simulink library "sm_motor_grader_lib"  (R2026a)
settings: Solver=VariableStepAuto
undefined symbols (not defined in the file): activeTestCmds, Art, Center, Circle, Driver, HMPST, LiftL, LiftR, LnL, LnR, Loads, Maneuver, motGradParams, Pin, RFL, RFR, RRL, RRR, SceneData, Side, Sphere, StrL, StrR, Tilt, X, Y, Z
libraries: sm_lib x219, nesl_utility x134, fl_lib x53, $bdroot x24, cvt_powertrain_lib x6, simulink_extras x5, grid_element x4, simulink x3, cvt_powertrain_lib_vnts x3, Driver_Long_Lat_Stanley x1, Maneuver_Get_Pose x1, SignalEditorBlockLib x1
(part 1 of 13)
Description:
  | Copyright 2025-2026 The MathWorks, Inc.
settings Model: Creator=smiller  LastModifiedBy=smiller

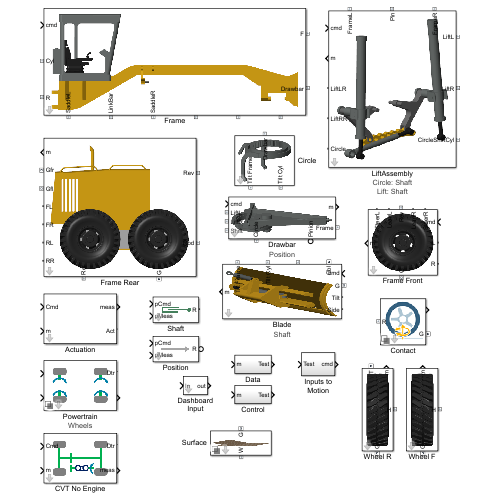
[thumbnail: Simulink's stored preview of the top-level diagram]
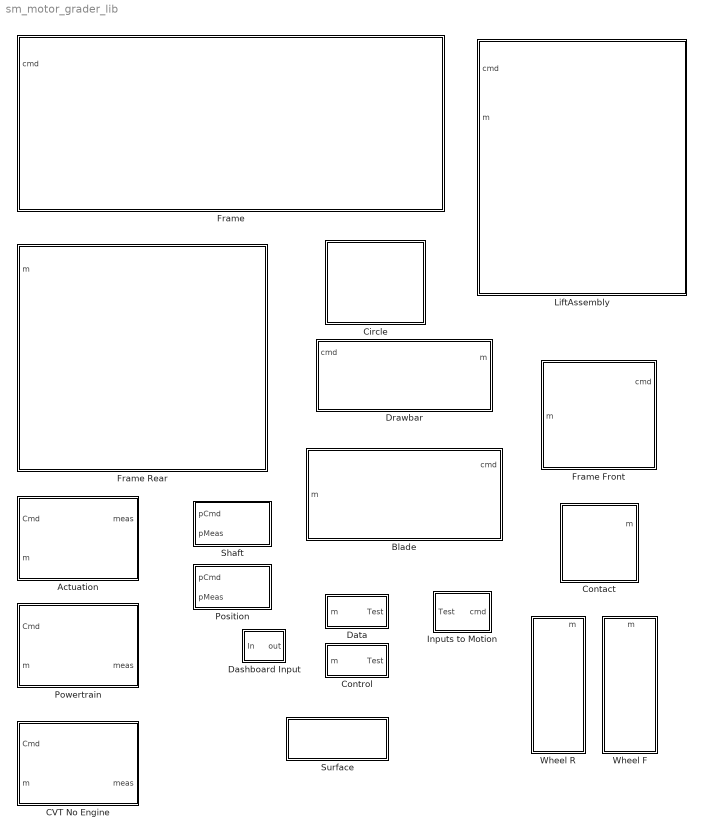
== system sm_motor_grader_lib ==
  Actuation : Subsystem  VariantControl=Actuation  mask{popup_actuator_model=Position, popup_actuator_model_lift=Shaft}
      mask prompts: popup_actuator_model "Actuation Mode"; popup_actuator_model_lift "Actuation Mode Lift"
      mask init:
      | bh = gcb;
      | modestr = get_param(bh,'popup_actuator_model');
      | set_param([bh '/Actuator Tilt'],'LabelModeActiveChoice',modestr)
      | set_param([bh '/Actuator Shift'],'LabelModeActiveChoice',modestr)
      | set_param([bh '/Actuator Articulation'],'LabelModeActiveChoice',modestr)
      | set_param([bh '/Actuator Circle'],'LabelModeActiveChoice',modestr)
      | set_param([bh '/Actuator SteerL'],'LabelModeActiveChoice',modestr)
      | set_param([bh '/Actuator SteerR'],'LabelModeActiveChoice',modestr)
      | set_param([bh '/Actuator LeanL'],'LabelModeActiveChoice',modestr)
      | set_param([bh '/Actuator LeanR'],'LabelModeActiveChoice',modestr)
      | set_param([bh '/Actuator Pinion'],'LabelModeActiveChoice',modestr)
      | 
      | liftmodestr = get_param(bh,'popup_actuator_model_lift');
      | set_param([bh '/Actuator LiftL'],'LabelModeActiveChoice',liftmodestr)
      | set_param([bh '/Actuator LiftR'],'LabelModeActiveChoice',liftmodestr)
      mask TypeOptions popup_actuator_model: Position | Shaft
      mask TypeOptions popup_actuator_model_lift: Position | Shaft
  Blade : Subsystem  mask{popup_actuator_model=Shaft, popup_blade_ground_contact=Loads}
      mask prompts: popup_actuator_model "Actuation Mode"; popup_blade_ground_contact "Blade Ground Contact"
      mask init:
      | bh = gcb;
      | if(strcmp(get_param(bh,'popup_actuator_model'),'Shaft'))
      |     set_param([bh '/Tilt Actuator'],'popup_actuator_model','Shaft')
      |     set_param([bh '/Shift Actuator'],'popup_actuator_model','Shaft')
      | else
      |     set_param([bh '/Tilt Actuator'],'popup_actuator_model','Position')
      |     set_param([bh '/Shift Actuator'],'popup_actuator_model','Position')
      | end
      settings: AttributesFormatString=%<popup_actuator_model>  PortSchema="{\"entries\":[{\"content\":{\"sides\":[{\"content\":{\"connectorIds\":[\"In1\",\"LConn1\",\"LConn2\",\"LConn3\"]},\"type\":\"ConnectorPlacement.EquallySpacedRectSide\",\"uuid\":\"64dbd0ba-121a-468c-87f8-2fede28d7949\"},{\"content\":{\"connectorIds\":[\"Out1\"],\"side\":\"RIGHT\"},\"type\":\"ConnectorPlacement.EquallySpacedRectSide\",\"uuid\":\"d521fda1-87cd-4ba3-938c-38986a441e94\"},{\"content\":{\"connectorIds\":[\"LConn4\",\"LConn5\",\"LConn6\",\"LConn7\"],\"side\":\"TOP\"},\"type\":\"ConnectorPlacement.EquallySpacedRectSide\",\"uuid\":\"c03a1403-e105-4f6f-8c6b-d646839b846b\"}]},\"type\":\"ConnectorPlacement.EquallySpacedConnector\",\"uuid\":\"70598b05-b8b5-4d67-bbf4-55a5797dbb69\"}],\"packageUris\":[\"http://schema.mathworks.com/mf0/Connector/R2020b\"],\"version\":\"1.0\"}"
      mask TypeOptions popup_actuator_model: Position | Shaft
      mask TypeOptions popup_blade_ground_contact: Blade/popup_blade_ground_contact
      mask Display: image('sm_motor_grader_moldboard_IMAGE.png')
  CVT No Engine : Subsystem  VariantControl=CVT
      settings: PortSchema="{\"entries\":[{\"content\":{\"sides\":[{\"content\":{\"connectorIds\":[\"In1\",\"In2\"]},\"type\":\"ConnectorPlacement.EquallySpacedRectSide\",\"uuid\":\"b0ddd375-51b8-44b6-b073-16b56860cf73\"},{\"content\":{\"connectorIds\":[\"RConn1\",\"Out1\"],\"side\":\"RIGHT\"},\"type\":\"ConnectorPlacement.EquallySpacedRectSide\",\"uuid\":\"f6b94886-5d75-4a34-bd54-ed8eca8a2f91\"},{\"content\":{\"side\":\"TOP\"},\"type\":\"ConnectorPlacement.EquallySpacedRectSide\",\"uuid\":\"a9bdb5f3-5bc9-4293-95f7-be33271ad817\"}]},\"type\":\"ConnectorPlacement.EquallySpacedConnector\",\"uuid\":\"99647ee7-7b0f-4a9d-8234-cdeac05b9707\"}],\"packageUris\":[\"http://schema.mathworks.com/mf0/Connector/R2020b\"],\"version\":\"1.0\"}"
      mask Display: image('ssc_4whl_powertrain_cvt.png')
  Circle : Subsystem
      settings: PortSchema="{\"entries\":[{\"content\":{\"sides\":[{\"content\":{},\"type\":\"ConnectorPlacement.EquallySpacedRectSide\",\"uuid\":\"63ab4a23-8b89-415d-877f-feb881a061f1\"},{\"content\":{\"side\":\"RIGHT\"},\"type\":\"ConnectorPlacement.EquallySpacedRectSide\",\"uuid\":\"0092ed81-5b75-47ad-b9e7-41c464aec9e6\"},{\"content\":{\"connectorIds\":[\"LConn1\"],\"side\":\"TOP\"},\"type\":\"ConnectorPlacement.EquallySpacedRectSide\",\"uuid\":\"752d188f-c013-4e13-8b29-1d347d2a3863\"},{\"content\":{\"connectorIds\":[\"RConn1\",\"RConn2\"],\"side\":\"BOTTOM\"},\"type\":\"ConnectorPlacement.EquallySpacedRectSide\",\"uuid\":\"b80fa618-c4c3-4c2f-8b58-79928366cbe4\"}]},\"type\":\"ConnectorPlacement.EquallySpacedConnector\",\"uuid\":\"1b957d24-5c42-454c-a11d-5e6b523a4d4e\"}],\"packageUris\":[\"http://schema.mathworks.com/mf0/Connector/R2020b\"],\"version\":\"1.0\"}"
      mask Display: image('sm_motor_grader_circle_IMAGE.png')
  Contact : Subsystem  Variant=on  VariantControlMode=label  VariantControl=Sphere  LabelModeActiveChoice=Magic Formula
  Control : Subsystem  VariantControl=Control
  Dashboard Input : Subsystem  mask{upper_bound=0, lower_bound=motGradParams.articulation.lowerBound, U0=motGradParams.articulation.initPos, tfilt=0.1}
      mask prompts: upper_bound "Upper Bound"; lower_bound "Lower Bound"; U0 "SimulinkBlocks:simulink_extras:InitialInput_MP"; tfilt "Filter Constant"
      mask TypeOptions U0:
      | Transfer Fcn
      | (with initial outputs)/U0 | Transfer Fcn
      | (with initial outputs)/Y0
      mask DialogControl U0 Prompt: Initial input:
  Data : Subsystem  VariantControl=Data
  Drawbar : Subsystem  mask{popup_actuator_model=Position}
      mask prompts: popup_actuator_model "Actuation Mode"
      mask init:
      | bh = gcb;
      | if(strcmp(get_param(bh,'popup_actuator_model'),'Shaft'))
      |     set_param([bh '/Actuator'],'LabelModeActiveChoice','Shaft')
      | else
      |     set_param([bh '/Actuator'],'LabelModeActiveChoice','Position')
      | end
      settings: AttributesFormatString=%<popup_actuator_model>  PortSchema="{\"entries\":[{\"content\":{\"sides\":[{\"content\":{\"connectorIds\":[\"In1\",\"LConn1\",\"LConn2\",\"LConn3\"]},\"type\":\"ConnectorPlacement.EquallySpacedRectSide\",\"uuid\":\"7234e91a-ed4b-4098-8d23-6b77775b5b7f\"},{\"content\":{\"connectorIds\":[\"Out1\",\"RConn1\"],\"side\":\"RIGHT\"},\"type\":\"ConnectorPlacement.EquallySpacedRectSide\",\"uuid\":\"48f806ee-3ea7-460b-b9fa-1f56f5dd994a\"},{\"content\":{\"side\":\"TOP\"},\"type\":\"ConnectorPlacement.EquallySpacedRectSide\",\"uuid\":\"5b9f253b-2dbf-4601-908f-7111d138ba6e\"},{\"content\":{\"connectorIds\":[\"RConn2\",\"RConn3\"],\"side\":\"BOTTOM\"},\"type\":\"ConnectorPlacement.EquallySpacedRectSide\",\"uuid\":\"9be04b94-2c6d-44c4-9c03-8c052620d49b\"}]},\"type\":\"ConnectorPlacement.EquallySpacedConnector\",\"uuid\":\"9d0450f6-732d-46a7-b755-37fed4fce1e3\"}],\"packageUris\":[\"http://schema.mathworks.com/mf0/Connector/R2020b\"],\"version\":\"1.0\"}"
      mask TypeOptions popup_actuator_model: Position | Shaft
      mask Display: image('sm_motor_grader_drawbar_IMAGE.png')
  Frame : Subsystem
      settings: PortSchema="{\"entries\":[{\"content\":{\"sides\":[{\"content\":{\"connectorIds\":[\"In1\",\"LConn1\",\"LConn2\"]},\"type\":\"ConnectorPlacement.EquallySpacedRectSide\",\"uuid\":\"b4e4171d-0284-478f-93eb-e40a965869bd\"},{\"content\":{\"connectorIds\":[\"RConn1\",\"RConn2\"],\"side\":\"RIGHT\"},\"type\":\"ConnectorPlacement.EquallySpacedRectSide\",\"uuid\":\"a326bb83-43f6-4b0d-ba21-f055f0976929\"},{\"content\":{\"side\":\"TOP\"},\"type\":\"ConnectorPlacement.EquallySpacedRectSide\",\"uuid\":\"b7d1be37-3d49-41f6-8566-6d4da5b1cd99\"},{\"content\":{\"connectorIds\":[\"RConn3\",\"RConn4\",\"RConn5\",\"RConn6\",\"RConn7\",\"RConn8\"],\"side\":\"BOTTOM\"},\"type\":\"ConnectorPlacement.EquallySpacedRectSide\",\"uuid\":\"50e3951f-3737-46e1-aff9-2ccd4ba65e65\"}]},\"type\":\"ConnectorPlacement.EquallySpacedConnector\",\"uuid\":\"94325d30-52dd-4a6f-8a1a-f56bc213c0cf\"}],\"packageUris\":[\"http://schema.mathworks.com/mf0/Connector/R2020b\"],\"version\":\"1.0\"}"
      mask Display: image('sm_motor_grader_frameCab_IMAGE.png')
  Frame Front : Subsystem  mask{popup_actuator_model=Shaft, popup_ground_contact=Sphere}
      mask prompts: popup_actuator_model "Actuation Mode"; popup_ground_contact "Ground Contact"
      mask init:
      | bh = gcb;
      | if(strcmp(get_param(bh,'popup_actuator_model'),'Shaft'))
      |     set_param([bh '/Lean Cylinder L'],'popup_actuator_model','Shaft')
      |     set_param([bh '/Lean Cylinder R'],'popup_actuator_model','Shaft')
      |     set_param([bh '/Steer Cylinder L'],'popup_actuator_model','Shaft')
      |     set_param([bh '/Steer Cylinder R'],'popup_actuator_model','Shaft')
      | else
      |     set_param([bh '/Lean Cylinder L'],'popup_actuator_model','Position')
      |     set_param([bh '/Lean Cylinder R'],'popup_actuator_model','Position')
      |     set_param([bh '/Steer Cylinder L'],'popup_actuator_model','Position')
      |     set_param([bh '/Steer Cylinder R'],'popup_actuator_model','Position')
      | end
      settings: PortSchema="{\"entries\":[{\"content\":{\"sides\":[{\"content\":{\"connectorIds\":[\"In1\",\"LConn1\",\"LConn2\"]},\"type\":\"ConnectorPlacement.EquallySpacedRectSide\",\"uuid\":\"d719529f-17dc-4c69-a89e-e71c8b487632\"},{\"content\":{\"connectorIds\":[\"Out1\"],\"side\":\"RIGHT\"},\"type\":\"ConnectorPlacement.EquallySpacedRectSide\",\"uuid\":\"e7fa06bf-1a63-484a-b998-aaa1bdc34664\"},{\"content\":{\"connectorIds\":[\"LConn3\",\"LConn4\",\"LConn5\",\"LConn6\",\"LConn7\"],\"side\":\"TOP\"},\"type\":\"ConnectorPlacement.EquallySpacedRectSide\",\"uuid\":\"3b968ecd-8edf-4595-9577-41521836e52d\"},{\"content\":{\"connectorIds\":[\"RConn1\"],\"side\":\"BOTTOM\"},\"type\":\"ConnectorPlacement.EquallySpacedRectSide\",\"uuid\":\"998a1490-38ee-4f90-9f0c-64c247eb2ef3\"}]},\"type\":\"ConnectorPlacement.EquallySpacedConnector\",\"uuid\":\"66e6443c-e818-4a0b-88cc-b534e33fe9c1\"}],\"packageUris\":[\"http://schema.mathworks.com/mf0/Connector/R2020b\"],\"version\":\"1.0\"}"
      mask TypeOptions popup_actuator_model: Position | Shaft
      mask TypeOptions popup_ground_contact: Wheel FL/popup_ground_contact | Wheel FR/popup_ground_contact
      mask Display: image('sm_motor_grader_frameFront_IMAGE.png')
  Frame Rear : Subsystem  mask{popup_ground_contact=Sphere}
      mask prompts: popup_ground_contact "Ground Contact"
      settings: PortSchema="{\"entries\":[{\"content\":{\"sides\":[{\"content\":{\"connectorIds\":[\"LConn1\",\"LConn2\"]},\"type\":\"ConnectorPlacement.EquallySpacedRectSide\",\"uuid\":\"e776eb69-fe07-42f6-973c-e6579d9bb0af\"},{\"content\":{\"connectorIds\":[\"Out1\",\"RConn1\",\"RConn2\",\"RConn3\",\"RConn4\",\"RConn5\",\"RConn6\"],\"side\":\"RIGHT\"},\"type\":\"ConnectorPlacement.EquallySpacedRectSide\",\"uuid\":\"308f9881-db51-4dcf-ba81-b3094ed7176e\"},{\"content\":{\"side\":\"TOP\"},\"type\":\"ConnectorPlacement.EquallySpacedRectSide\",\"uuid\":\"d5cd9905-25fb-439a-a908-e078aef10600\"},{\"content\":{\"connectorIds\":[\"RConn7\",\"RConn8\"],\"side\":\"BOTTOM\"},\"type\":\"ConnectorPlacement.EquallySpacedRectSide\",\"uuid\":\"fcfd5f0a-595a-4c14-8789-0bf7c20d2a5f\"}]},\"type\":\"ConnectorPlacement.EquallySpacedConnector\",\"uuid\":\"05355ae5-5c0f-4ba9-8d92-15da5bd4be6c\"}],\"packageUris\":[\"http://schema.mathworks.com/mf0/Connector/R2020b\"],\"version\":\"1.0\"}"
      mask TypeOptions popup_ground_contact: Wheel FL/popup_ground_contact | Wheel FR/popup_ground_contact | Wheel RL/popup_ground_contact | Wheel RR/popup_ground_contact
      mask Display: image('sm_motor_grader_frameRear_IMAGE.png')
  Inputs to Motion : Subsystem
  LiftAssembly : Subsystem  mask{popup_actuator_model=Shaft, popup_actuator_model_lift=Shaft, popup_initial_hole=Center}
      mask prompts: popup_actuator_model "Actuation Mode"; popup_actuator_model_lift "Actuation Mode Lift"; popup_initial_hole "Link Bar Initial Hole"
      mask init:
      | bh = gcb;
      | modestr = get_param(bh,'popup_actuator_model');
      | set_param([bh '/Circle Shift'],'popup_actuator_model',modestr)
      | 
      | liftmodestr = get_param(bh,'popup_actuator_model_lift');
      | set_param([bh '/Saddle L'],'popup_actuator_model',liftmodestr)
      | set_param([bh '/Saddle R'],'popup_actuator_model',liftmodestr)
      settings: PortSchema="{\"entries\":[{\"content\":{\"sides\":[{\"content\":{\"connectorIds\":[\"In1\",\"Out1\",\"LConn1\",\"LConn2\",\"LConn3\"]},\"type\":\"ConnectorPlacement.EquallySpacedRectSide\",\"uuid\":\"75f9baa5-7280-4f07-a363-ed0a46c03729\"},{\"content\":{\"connectorIds\":[\"RConn1\",\"RConn2\",\"RConn3\"],\"side\":\"RIGHT\"},\"type\":\"ConnectorPlacement.EquallySpacedRectSide\",\"uuid\":\"3ff26dde-6195-402e-b2bb-6b31a89f247a\"},{\"content\":{\"connectorIds\":[\"LConn4\",\"LConn5\",\"LConn6\"],\"side\":\"TOP\"},\"type\":\"ConnectorPlacement.EquallySpacedRectSide\",\"uuid\":\"71d0d382-4fbb-4984-aa84-52a20f8bddb0\"}]},\"type\":\"ConnectorPlacement.EquallySpacedConnector\",\"uuid\":\"07638312-eb37-4222-9751-dc3e74f2a474\"}],\"packageUris\":[\"http://schema.mathworks.com/mf0/Connector/R2020b\"],\"version\":\"1.0\"}"
      settings: AttributesFormatString=|
      | Circle: %<popup_actuator_model>
      | Lift: %<popup_actuator_model_lift>
      mask TypeOptions popup_actuator_model: Position | Shaft
      mask TypeOptions popup_actuator_model_lift: Position | Shaft
      mask TypeOptions popup_initial_hole: LinkBar/popup_initial_hole
      mask Display: image('sm_motor_grader_liftAssy_IMAGE.png')
  Position : Subsystem  VariantControl=Position
      mask Display: image('sm_motor_grader_actuation_Position_IMAGE.png')
  Powertrain : Subsystem  Variant=on  VariantControlMode=label  VariantControl=Powertrain  LabelModeActiveChoice=Torque4  mask{popup_powertrain_config=Wheels}
      mask prompts: popup_powertrain_config "Powertrain Configuration"
      mask init:
      | blk_h = gcb;
      | switch(get_param(blk_h,'popup_powertrain_config'))
      |     case('Wheels')
      |         set_param(blk_h,'LabelModeActiveChoice','Torque4');
      |     case('Driveline')
      |         set_param(blk_h,'LabelModeActiveChoice','Torque1');
      |     case('CVT Abstract')
      |         set_param(blk_h,'LabelModeActiveChoice','CVT');
      |         set_param([blk_h '/CVT/Transmission'],'LabelModeActiveChoice','Abstract');
      |     case('CVT Electrical')
      |         set_param(blk_h,'LabelModeActiveChoice','CVT');
      |         set_param([blk_h '/CVT/Transmission'],'LabelModeActiveChoice','Electrical');
      |     case('CVT Hydrostatic')
      |         set_param(blk_h,'LabelModeActiveChoice','CVT');
      |         set_param([blk_h '/CVT/Transmission'],'LabelModeActiveChoice','Hydrostatic');
      |     case('CVT Power Split HM')
      |         set_param(blk_h,'LabelModeActiveChoice','CVT');
      |         set_param([blk_h '/CVT/Transmission'],'LabelModeActiveChoice','Power_Split_HM');
      | end
      settings: AttributesFormatString=%<popup_powertrain_config>  PortSchema="{\"entries\":[{\"content\":{\"sides\":[{\"content\":{\"connectorIds\":[\"In1\",\"In2\"]},\"type\":\"ConnectorPlacement.EquallySpacedRectSide\",\"uuid\":\"b0ddd375-51b8-44b6-b073-16b56860cf73\"},{\"content\":{\"connectorIds\":[\"RConn1\",\"Out1\"],\"side\":\"RIGHT\"},\"type\":\"ConnectorPlacement.EquallySpacedRectSide\",\"uuid\":\"f6b94886-5d75-4a34-bd54-ed8eca8a2f91\"},{\"content\":{\"side\":\"TOP\"},\"type\":\"ConnectorPlacement.EquallySpacedRectSide\",\"uuid\":\"a9bdb5f3-5bc9-4293-95f7-be33271ad817\"}]},\"type\":\"ConnectorPlacement.EquallySpacedConnector\",\"uuid\":\"99647ee7-7b0f-4a9d-8234-cdeac05b9707\"}],\"packageUris\":[\"http://schema.mathworks.com/mf0/Connector/R2020b\"],\"version\":\"1.0\"}"
      mask TypeOptions popup_powertrain_config: Wheels | Driveline | CVT Abstract | CVT Electrical | CVT Hydrostatic | CVT Power Split HM
  Shaft : Subsystem  VariantControl=Shaft  mask{Kp=motGradParams.bladeTilt.propGain, Ki=motGradParams.bladeTilt.integral, Kd=motGradParams.bladeTilt.derivative, p_init=motGradParams.bladeTilt.initPos}
      mask prompts: Kp "Proportional Gain"; Ki "Integral Gain"; Kd "Derivative Gain"; p_init "Initial Position"
      mask Display: image('sm_motor_grader_actuation_Shaft_IMAGE.png')
  Surface : Subsystem  Variant=on  VariantControlMode=label  VariantControl=Grid  LabelModeActiveChoice=Bank  mask{popup_surface_type=Bank}
      mask prompts: popup_surface_type "Surface"
      mask init:
      | bh = gcb;
      | set_param(bh,'LabelModeActiveChoice',get_param(bh,'popup_surface_type'));
      mask TypeOptions popup_surface_type: Grid | Bank | Parked | Terrain
  Wheel F : Subsystem  mask{popup_ground_contact=Sphere, popup_leftright=Left}
      mask prompts: popup_ground_contact "Ground Contact"; popup_leftright "Left or Right"
      mask init:
      | bh = gcb;
      | set_param([bh '/Contact'],'LabelModeActiveChoice',get_param(bh,'popup_ground_contact'));
      | 
      | leftRight = get_param(bh,'popup_leftright');
      | side_lr = 0;
      | if(strcmpi(leftRight,'right'))
      |     side_lr = 1;
      | end
      settings: PortSchema="{\"entries\":[{\"content\":{\"sides\":[{\"content\":{\"connectorIds\":[\"LConn1\"]},\"type\":\"ConnectorPlacement.EquallySpacedRectSide\",\"uuid\":\"a2396ce2-0b10-4ac3-a1ec-372f9460b0ae\"},{\"content\":{\"side\":\"RIGHT\"},\"type\":\"ConnectorPlacement.EquallySpacedRectSide\",\"uuid\":\"bc399dab-ed7e-4e42-b626-ea0039165e7e\"},{\"content\":{\"connectorIds\":[\"Out1\"],\"side\":\"TOP\"},\"type\":\"ConnectorPlacement.EquallySpacedRectSide\",\"uuid\":\"15d89ddc-1aa5-4250-a204-7e514afbf964\"},{\"content\":{\"connectorIds\":[\"RConn1\"],\"side\":\"BOTTOM\"},\"type\":\"ConnectorPlacement.EquallySpacedRectSide\",\"uuid\":\"0e3863c0-9b5e-4093-9fa1-e5d7d0957fcd\"}]},\"type\":\"ConnectorPlacement.EquallySpacedConnector\",\"uuid\":\"b0026825-a0f7-4be5-bd6d-217e8c3590d5\"}],\"packageUris\":[\"http://schema.mathworks.com/mf0/Connector/R2020b\"],\"version\":\"1.0\"}"
      mask TypeOptions popup_ground_contact: Sphere | Point Cloud | Magic Formula
      mask TypeOptions popup_leftright: Left | Right
      mask Display: image('sm_motor_grader_actuator_tire_IMAGE.png')
  Wheel R : Subsystem  mask{popup_ground_contact=Sphere, popup_leftright=Left}
      mask prompts: popup_ground_contact "Ground Contact"; popup_leftright "Left or Right"
      mask init: same as sm_motor_grader_lib/Wheel F
      settings: PortSchema="{\"entries\":[{\"content\":{\"sides\":[{\"content\":{},\"type\":\"ConnectorPlacement.EquallySpacedRectSide\",\"uuid\":\"89ae7f7f-214f-46a4-a5eb-724a39bb80a0\"},{\"content\":{\"connectorIds\":[\"RConn1\"],\"side\":\"RIGHT\"},\"type\":\"ConnectorPlacement.EquallySpacedRectSide\",\"uuid\":\"543eaeb8-c3d6-4a28-93a8-4ee0452bf8f4\"},{\"content\":{\"connectorIds\":[\"LConn1\",\"Out1\"],\"side\":\"TOP\"},\"type\":\"ConnectorPlacement.EquallySpacedRectSide\",\"uuid\":\"e3b48660-4283-4eb0-87af-c87809de85ed\"},{\"content\":{\"connectorIds\":[\"RConn2\"],\"side\":\"BOTTOM\"},\"type\":\"ConnectorPlacement.EquallySpacedRectSide\",\"uuid\":\"a747ec4d-29c5-47e1-bb6d-f40774851901\"}]},\"type\":\"ConnectorPlacement.EquallySpacedConnector\",\"uuid\":\"be8b2801-2df3-46ac-8729-63aa4c1d31c6\"}],\"packageUris\":[\"http://schema.mathworks.com/mf0/Connector/R2020b\"],\"version\":\"1.0\"}"
      mask TypeOptions popup_ground_contact: Sphere | Point Cloud | Magic Formula
      mask TypeOptions popup_leftright: Left | Right
      mask Display: image('sm_motor_grader_actuator_tire_IMAGE.png')

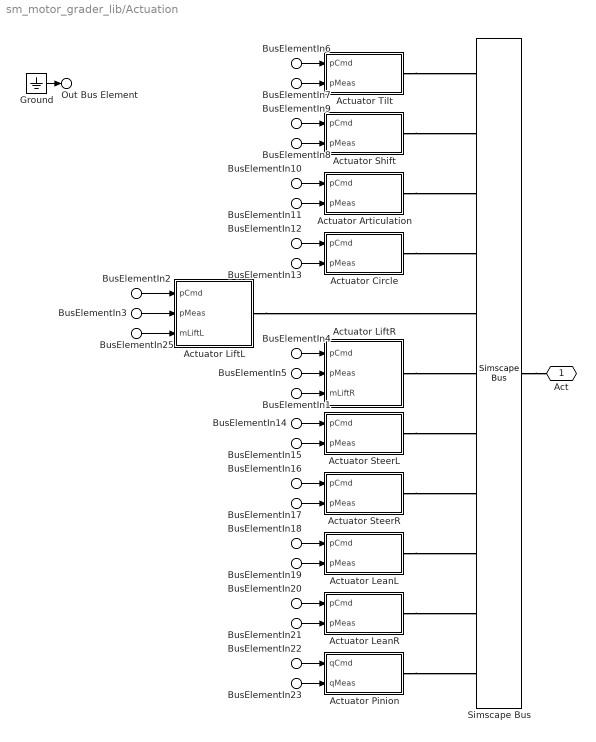
== system sm_motor_grader_lib/Actuation ==
  BusElementIn2 : Inport  PortName=Cmd  Element=pLiftL
  BusElementIn4 : Inport  PortName=Cmd  Element=pLiftR
  BusElementIn6 : Inport  PortName=Cmd  Element=pTilt
  BusElementIn9 : Inport  PortName=Cmd  Element=pShift
  BusElementIn10 : Inport  PortName=Cmd  Element=pArtic
  BusElementIn12 : Inport  PortName=Cmd  Element=pCircleShift
  BusElementIn14 : Inport  PortName=Cmd  Element=pSteerL
  BusElementIn16 : Inport  PortName=Cmd  Element=pSteerR
  BusElementIn18 : Inport  PortName=Cmd  Element=pLeanL
  BusElementIn20 : Inport  PortName=Cmd  Element=pLeanR
  BusElementIn22 : Inport  PortName=Cmd  Element=qCircle
  BusElementIn25 : Inport  PortName=Cmd  Element=mLiftL
  BusElementIn1 : Inport  PortName=Cmd  Element=mLiftR
  BusElementIn7 : Inport  Port=2  PortName=m  Element=Frame.Blade.Tilt.p
  BusElementIn8 : Inport  Port=2  PortName=m  Element=Frame.Blade.Shift.p
  BusElementIn3 : Inport  Port=2  PortName=m  Element=Frame.Lift.LiftL.p
  BusElementIn5 : Inport  Port=2  PortName=m  Element=Frame.Lift.LiftR.p
  BusElementIn13 : Inport  Port=2  PortName=m  Element=Frame.Lift.CircleShift.p
  BusElementIn23 : Inport  Port=2  PortName=m  Element=Frame.Drawbar.Circle.q
  BusElementIn11 : Inport  Port=2  PortName=m  Element=Artic.p
  BusElementIn15 : Inport  Port=2  PortName=m  Element=FrameF.SteerL.p
  BusElementIn17 : Inport  Port=2  PortName=m  Element=FrameF.SteerR.p
  BusElementIn19 : Inport  Port=2  PortName=m  Element=FrameF.LeanL.p
  BusElementIn21 : Inport  Port=2  PortName=m  Element=FrameF.LeanR.p
  Actuator Articulation : Subsystem  Variant=on  VariantControlMode=label  VariantControl=Actuator Articulation  LabelModeActiveChoice=Position
  Actuator Circle : Subsystem  Variant=on  VariantControlMode=label  VariantControl=Actuator Circle  LabelModeActiveChoice=Position
  Actuator LeanL : Subsystem  Variant=on  VariantControlMode=label  VariantControl=Actuator LeanL  LabelModeActiveChoice=Position
  Actuator LeanR : Subsystem  Variant=on  VariantControlMode=label  VariantControl=Actuator LeanR  LabelModeActiveChoice=Position
  Actuator LiftL : Subsystem  Variant=on  VariantControlMode=label  VariantControl=Actuator LiftL  LabelModeActiveChoice=Shaft
  Actuator LiftR : Subsystem  Variant=on  VariantControlMode=label  VariantControl=Actuator LiftR  LabelModeActiveChoice=Shaft
  Actuator Pinion : Subsystem  Variant=on  VariantControlMode=label  VariantControl=Actuator Pinion  LabelModeActiveChoice=Position
  Actuator Shift : Subsystem  Variant=on  VariantControlMode=label  VariantControl=Actuator Shift  LabelModeActiveChoice=Position
  Actuator SteerL : Subsystem  Variant=on  VariantControlMode=label  VariantControl=Actuator SteerL  LabelModeActiveChoice=Position
  Actuator SteerR : Subsystem  Variant=on  VariantControlMode=label  VariantControl=Actuator SteerR  LabelModeActiveChoice=Position
  Actuator Tilt : Subsystem  Variant=on  VariantControlMode=label  VariantControl=Actuator Tilt  LabelModeActiveChoice=Position
      settings: AttributesFormatString=%<LabelModeActiveChoice>
  Ground : Ground
  Simscape Bus : SimscapeBus  HierarchyStrings=Tilt;Side;Art;Circle;LiftL;LiftR;StrL;StrR;LnL;LnR;Pin
  Act : PMIOPort  Side=Right
  Out Bus Element : Outport  PortName=meas  Element=Actuator
  wires:
  BusElementIn6/1 -> Actuator Tilt/1(pCmd)
  BusElementIn7/1 -> Actuator Tilt/2(pMeas)
  BusElementIn9/1 -> Actuator Shift/1(pCmd)
  BusElementIn8/1 -> Actuator Shift/2(pMeas)
  BusElementIn10/1 -> Actuator Articulation/1(pCmd)
  BusElementIn11/1 -> Actuator Articulation/2(pMeas)
  BusElementIn12/1 -> Actuator Circle/1(pCmd)
  BusElementIn13/1 -> Actuator Circle/2(pMeas)
  BusElementIn14/1 -> Actuator SteerL/1(pCmd)
  BusElementIn15/1 -> Actuator SteerL/2(pMeas)
  BusElementIn16/1 -> Actuator SteerR/1(pCmd)
  BusElementIn17/1 -> Actuator SteerR/2(pMeas)
  BusElementIn18/1 -> Actuator LeanL/1(pCmd)
  BusElementIn19/1 -> Actuator LeanL/2(pMeas)
  BusElementIn20/1 -> Actuator LeanR/1(pCmd)
  BusElementIn21/1 -> Actuator LeanR/2(pMeas)
  BusElementIn22/1 -> Actuator Pinion/1(qCmd)
  BusElementIn23/1 -> Actuator Pinion/2(qMeas)
  BusElementIn25/1 -> Actuator LiftL/3(mLiftL)
  BusElementIn3/1 -> Actuator LiftL/2(pMeas)
  BusElementIn2/1 -> Actuator LiftL/1(pCmd)
  BusElementIn4/1 -> Actuator LiftR/1(pCmd)
  BusElementIn5/1 -> Actuator LiftR/2(pMeas)
  BusElementIn1/1 -> Actuator LiftR/3(mLiftR)
  Ground/1 -> Out Bus Element/1
  connections:
  Simscape Bus/RConn1 -- Act/RConn1
  Actuator Tilt/RConn1 -- Simscape Bus/LConn1
  Actuator Shift/RConn1 -- Simscape Bus/LConn2
  Actuator Articulation/RConn1 -- Simscape Bus/LConn3
  Actuator Circle/RConn1 -- Simscape Bus/LConn4
  Actuator LiftL/RConn1 -- Simscape Bus/LConn5
  Actuator LiftR/RConn1 -- Simscape Bus/LConn6
  Actuator SteerL/RConn1 -- Simscape Bus/LConn7
  Actuator SteerR/RConn1 -- Simscape Bus/LConn8
  Actuator LeanL/RConn1 -- Simscape Bus/LConn9
  Actuator LeanR/RConn1 -- Simscape Bus/LConn10
  Actuator Pinion/RConn1 -- Simscape Bus/LConn11

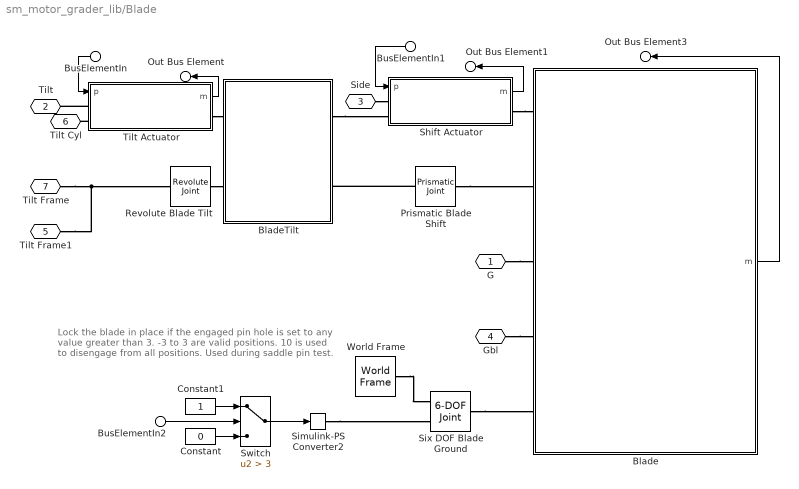
== system sm_motor_grader_lib/Blade ==
  note: Lock the blade in place if the engaged pin hole is set to any value greater than 3. -3 to 3 are valid positions. 10 is used to disengage from all positions. Used during saddle pin test.
  BusElementIn : Inport  PortName=cmd  Element=pTilt
  BusElementIn1 : Inport  PortName=cmd  Element=pShift
  BusElementIn2 : Inport  PortName=cmd  Element=nHoleLink
  Blade : Subsystem  mask{popup_blade_ground_contact=Loads}
      mask prompts: popup_blade_ground_contact "Blade Ground Contact"
      mask TypeOptions popup_blade_ground_contact: Ground Forces/popup_blade_ground_contact
      mask Display: image('sm_motor_grader_blade_IMAGE.png')
  BladeTilt : Subsystem
      mask Display: image('sm_motor_grader_bladeTilt_IMAGE.png')
  Constant : Constant  Value=0
  Constant1 : Constant
  Prismatic Blade Shift : sm_lib/Joints/Prismatic Joint  JointMode=Normal  CompositeWrenchDir=FollowerOnBase  CompositeWrenchFrame=BaseFrame  SenseConstraintForce=off  SenseConstraintTorque=off  SenseTotalForce=off  SenseTotalTorque=off  PositionTargetSpecify=off  PositionTargetPriority=High  PositionTargetValue=0  PositionTargetValueUnits=m  VelocityTargetSpecify=off  VelocityTargetPriority=High  VelocityTargetValue=0  VelocityTargetValueUnits=m/s  EquilibriumPosition=0  EquilibriumPositionUnits=m  SpringStiffness=0  SpringStiffnessUnits=N/m  DampingCoefficient=motGradParams.bladeSideShift.damping  DampingCoefficientUnits=N/(m/s)  LowerLimitSpecify=off  LowerLimitBound=-1  LowerLimitBoundUnits=m  LowerLimitStiffness=1e6  LowerLimitStiffnessUnits=N/m  LowerLimitDamping=1e3  LowerLimitDampingUnits=N/(m/s)  LowerLimitTransitionRegionWidth=1e-4  LowerLimitTransitionRegionWidthUnits=m  UpperLimitSpecify=off  UpperLimitBound=1  UpperLimitBoundUnits=m  UpperLimitStiffness=1e6  UpperLimitStiffnessUnits=N/m  UpperLimitDamping=1e3  UpperLimitDampingUnits=N/(m/s)  UpperLimitTransitionRegionWidth=1e-4  UpperLimitTransitionRegionWidthUnits=m  TorqueActuationMode=NoTorque  MotionActuationMode=ComputedMotion  SensePosition=off  SenseVelocity=off  SenseAcceleration=off  SenseTorqueForce=off  SenseLowerLimitTorqueForce=off  SenseUpperLimitTorqueForce=off
  Revolute Blade Tilt : sm_lib/Joints/Revolute Joint  JointMode=Normal  CompositeWrenchDir=FollowerOnBase  CompositeWrenchFrame=BaseFrame  SenseConstraintForce=off  SenseConstraintTorque=off  SenseTotalForce=off  SenseTotalTorque=off  PositionTargetSpecify=off  PositionTargetPriority=High  PositionTargetValue=0  PositionTargetValueUnits=deg  VelocityTargetSpecify=off  VelocityTargetPriority=High  VelocityTargetValue=0  VelocityTargetValueUnits=deg/s  EquilibriumPosition=0  EquilibriumPositionUnits=deg  SpringStiffness=0  SpringStiffnessUnits=N*m/deg  DampingCoefficient=motGradParams.revDampingCoeff  DampingCoefficientUnits=N*m/(deg/s)  LowerLimitSpecify=off  LowerLimitBound=-90  LowerLimitBoundUnits=deg  LowerLimitStiffness=1e4  LowerLimitStiffnessUnits=N*m/deg  LowerLimitDamping=10  LowerLimitDampingUnits=N*m/(deg/s)  LowerLimitTransitionRegionWidth=0.1  LowerLimitTransitionRegionWidthUnits=deg  UpperLimitSpecify=off  UpperLimitBound=90  UpperLimitBoundUnits=deg  UpperLimitStiffness=1e4  UpperLimitStiffnessUnits=N*m/deg  UpperLimitDamping=10  UpperLimitDampingUnits=N*m/(deg/s)  UpperLimitTransitionRegionWidth=0.1  UpperLimitTransitionRegionWidthUnits=deg  TorqueActuationMode=NoTorque  MotionActuationMode=ComputedMotion  SensePosition=off  SenseVelocity=off  SenseAcceleration=off  SenseTorqueForce=off  SenseLowerLimitTorqueForce=off  SenseUpperLimitTorqueForce=off
  Shift Actuator : Subsystem  mask{popup_actuator_model=Shaft}
      mask prompts: popup_actuator_model "Actuation Mode"
      mask init: same as sm_motor_grader_lib/Drawbar
      settings: AttributesFormatString=%<popup_actuator_model>
      mask TypeOptions popup_actuator_model: Position | Shaft
      mask Display:
      | bh = gcb;
      | if(strcmp(get_param(bh,'popup_actuator_model'),'Position'))
      |     image('sm_motor_grader_actuator_intfPosition_IMAGE.png')
      | else
      |     image('sm_motor_grader_actuator_intfShaft_IMAGE.png')
      | end
  Simulink-PS Converter2 : nesl_utility/Simulink-PS Converter  PhysicalDomain=network_engine_domain  SubClassName=ps_input  LeftPortType=input  RightPortType=output  PseudoPeriodic=off  Frequencies=[]  NoiseDistribution=none  NoiseParameters=[]  Unit=1  AffineConversion=off  FilteringAndDerivatives=provide  SimscapeFilterOrder=1  InputFilterTimeConstant=0.001  UdotUserProvided=0
  Six DOF Blade Ground : sm_lib/Joints/6-DOF Joint  JointMode=ProvidedByInput  CompositeWrenchDir=FollowerOnBase  CompositeWrenchFrame=BaseFrame  SenseConstraintForce=off  SenseConstraintTorque=off  SenseTotalForce=off  SenseTotalTorque=off  PxPositionTargetSpecify=off  PxPositionTargetPriority=High  PxPositionTargetValue=0  PxPositionTargetValueUnits=m  PxVelocityTargetSpecify=off  PxVelocityTargetPriority=High  PxVelocityTargetValue=0  PxVelocityTargetValueUnits=m/s  PxEquilibriumPosition=0  PxEquilibriumPositionUnits=m  PxSpringStiffness=0  PxSpringStiffnessUnits=N/m  PxDampingCoefficient=0  PxDampingCoefficientUnits=N/(m/s)  PxLowerLimitSpecify=off  PxLowerLimitBound=-1  PxLowerLimitBoundUnits=m  PxLowerLimitStiffness=1e6  PxLowerLimitStiffnessUnits=N/m  PxLowerLimitDamping=1e3  PxLowerLimitDampingUnits=N/(m/s)  PxLowerLimitTransitionRegionWidth=1e-4  PxLowerLimitTransitionRegionWidthUnits=m  PxUpperLimitSpecify=off  PxUpperLimitBound=1  PxUpperLimitBoundUnits=m  PxUpperLimitStiffness=1e6  PxUpperLimitStiffnessUnits=N/m  PxUpperLimitDamping=1e3  PxUpperLimitDampingUnits=N/(m/s)  PxUpperLimitTransitionRegionWidth=1e-4  PxUpperLimitTransitionRegionWidthUnits=m  PxTorqueActuationMode=NoTorque  PxMotionActuationMode=ComputedMotion  PxSensePosition=off  PxSenseVelocity=off  PxSenseAcceleration=off  PxSenseTorqueForce=off  PxSenseLowerLimitTorqueForce=off  PxSenseUpperLimitTorqueForce=off  PyPositionTargetSpecify=off  PyPositionTargetPriority=High  PyPositionTargetValue=0  PyPositionTargetValueUnits=m  PyVelocityTargetSpecify=off  PyVelocityTargetPriority=High  PyVelocityTargetValue=0  PyVelocityTargetValueUnits=m/s  PyEquilibriumPosition=0  PyEquilibriumPositionUnits=m  PySpringStiffness=0  PySpringStiffnessUnits=N/m  PyDampingCoefficient=0  PyDampingCoefficientUnits=N/(m/s)  PyLowerLimitSpecify=off  PyLowerLimitBound=-1  PyLowerLimitBoundUnits=m  PyLowerLimitStiffness=1e6  PyLowerLimitStiffnessUnits=N/m  PyLowerLimitDamping=1e3  PyLowerLimitDampingUnits=N/(m/s)  PyLowerLimitTransitionRegionWidth=1e-4  PyLowerLimitTransitionRegionWidthUnits=m  PyUpperLimitSpecify=off  PyUpperLimitBound=1  PyUpperLimitBoundUnits=m  PyUpperLimitStiffness=1e6  PyUpperLimitStiffnessUnits=N/m  PyUpperLimitDamping=1e3  PyUpperLimitDampingUnits=N/(m/s)  PyUpperLimitTransitionRegionWidth=1e-4  PyUpperLimitTransitionRegionWidthUnits=m  PyTorqueActuationMode=NoTorque  PyMotionActuationMode=ComputedMotion  PySensePosition=off  PySenseVelocity=off  PySenseAcceleration=off  PySenseTorqueForce=off  PySenseLowerLimitTorqueForce=off  PySenseUpperLimitTorqueForce=off  PzPositionTargetSpecify=off  PzPositionTargetPriority=High  PzPositionTargetValue=0  PzPositionTargetValueUnits=m  PzVelocityTargetSpecify=off  PzVelocityTargetPriority=High  PzVelocityTargetValue=0  PzVelocityTargetValueUnits=m/s  PzEquilibriumPosition=0  PzEquilibriumPositionUnits=m  PzSpringStiffness=0  PzSpringStiffnessUnits=N/m  PzDampingCoefficient=0  PzDampingCoefficientUnits=N/(m/s)  PzLowerLimitSpecify=off  PzLowerLimitBound=-1  PzLowerLimitBoundUnits=m  PzLowerLimitStiffness=1e6  PzLowerLimitStiffnessUnits=N/m  PzLowerLimitDamping=1e3  PzLowerLimitDampingUnits=N/(m/s)  PzLowerLimitTransitionRegionWidth=1e-4  PzLowerLimitTransitionRegionWidthUnits=m  PzUpperLimitSpecify=off  PzUpperLimitBound=1  PzUpperLimitBoundUnits=m  PzUpperLimitStiffness=1e6  PzUpperLimitStiffnessUnits=N/m  PzUpperLimitDamping=1e3  PzUpperLimitDampingUnits=N/(m/s)  PzUpperLimitTransitionRegionWidth=1e-4  PzUpperLimitTransitionRegionWidthUnits=m  PzTorqueActuationMode=NoTorque  PzMotionActuationMode=ComputedMotion  PzSensePosition=off  PzSenseVelocity=off  PzSenseAcceleration=off  PzSenseTorqueForce=off  PzSenseLowerLimitTorqueForce=off  PzSenseUpperLimitTorqueForce=off  SphPositionTargetSpecify=off  SphPositionTargetPriority=High  SphPositionTargetRotationMethod=None  SphPositionTargetFollAlignAxisA=+X  SphPositionTargetBaseAlignAxisA=+Y  SphPositionTargetFollAlignAxisB=+Y  SphPositionTargetBaseAlignAxisB=+Z  SphPositionTargetRotationStandardAxis=+Z  SphPositionTargetRotationAngle=0  SphPositionTargetRotationAngleUnits=deg  SphPositionTargetRotationArbitraryAxis=[0 0 1]  SphPositionTargetRotationSequenceAxes=FollowerAxes  SphPositionTargetRotationSequence=XYX  SphPositionTargetRotationSequenceAngles=[0 0 0]  SphPositionTargetRotationSequenceAnglesUnits=deg  SphPositionTargetRotationMatrix=[1 0 0;0 1 0;0 0 1]  SphPositionTargetQuaternion=[1 0 0 0]  SphVelocityTargetSpecify=off  SphVelocityTargetPriority=High  SphVelocityTargetValue=[0 0 0]  SphVelocityTargetValueUnits=deg/s  SphVelocityTargetInFollowerFrame=on  SphEqPosRotationMethod=None  SphEqPosFollAlignAxisA=+X  SphEqPosBaseAlignAxisA=+Y  SphEqPosFollAlignAxisB=+Y  SphEqPosBaseAlignAxisB=+Z  SphEqPosRotationStandardAxis=+Z  SphEqPosRotationAngle=0  SphEqPosRotationAngleUnits=deg  SphEqPosRotationArbitraryAxis=[0 0 1]  SphEqPosRotationSequenceAxes=FollowerAxes  SphEqPosRotationSequence=XYX  SphEqPosRotationSequenceAngles=[0 0 0]  SphEqPosRotationSequenceAnglesUnits=deg  SphEqPosRotationMatrix=[1 0 0;0 1 0;0 0 1]  SphEqPosQuaternion=[1 0 0 0]  SphSpringStiffness=0  SphSpringStiffnessUnits=N*m/deg  SphDampingCoefficient=0  SphDampingCoefficientUnits=N*m/(deg/s)  SphLowerLimitSpecify=off  SphLowerLimitBound=15  SphLowerLimitBoundUnits=deg  SphLowerLimitStiffness=1e4  SphLowerLimitStiffnessUnits=N*m/deg  SphLowerLimitDamping=10  SphLowerLimitDampingUnits=N*m/(deg/s)  SphLowerLimitTransitionRegionWidth=0.1  SphLowerLimitTransitionRegionWidthUnits=deg  SphUpperLimitSpecify=off  SphUpperLimitBound=45  SphUpperLimitBoundUnits=deg  SphUpperLimitStiffness=1e4  SphUpperLimitStiffnessUnits=N*m/deg  SphUpperLimitDamping=10  SphUpperLimitDampingUnits=N*m/(deg/s)  SphUpperLimitTransitionRegionWidth=0.1  SphUpperLimitTransitionRegionWidthUnits=deg  SphTorqueActuationMode=NoTorque  SphActuateTorqueX=off  SphActuateTorqueY=off  SphActuateTorqueZ=off  SphActuateTorque=off  SphActuationFrame=BaseFrame  SphSensePosition=off  SphSenseVelocityX=off  SphSenseVelocityY=off  SphSenseVelocityZ=off  SphSenseVelocity=off  SphSenseAccelerationX=off  SphSenseAccelerationY=off  SphSenseAccelerationZ=off  SphSenseAcceleration=off  SphSenseLowerLimitTorqueMag=off  SphSenseUpperLimitTorqueMag=off  SphSensingFrame=BaseFrame
  Switch : Switch  Criteria=u2 > Threshold  Threshold=3  SaturateOnIntegerOverflow=off  InputSameDT=off
  Tilt Actuator : Subsystem  mask{popup_actuator_model=Shaft}
      mask prompts: popup_actuator_model "Actuation Mode"
      mask init: same as sm_motor_grader_lib/Drawbar
      settings: AttributesFormatString=%<popup_actuator_model>
      mask TypeOptions popup_actuator_model: Position | Shaft
      mask Display:
      | bh = gcb;
      | if(strcmp(get_param(bh,'popup_actuator_model'),'Position'))
      |     image('sm_motor_grader_actuator_intfPosition_IMAGE.png')
      | else
      |     image('sm_motor_grader_actuator_intfShaft_IMAGE.png')
      | end
  World Frame : sm_lib/Frames and Transforms/World Frame
  G : PMIOPort  Side=Left
  Tilt : PMIOPort  Port=2  Side=Left
  Side : PMIOPort  Port=3  Side=Left
  Gbl : PMIOPort  Port=4  Side=Left
  Tilt Frame1 : PMIOPort  Port=5  Side=Left
  Tilt Cyl : PMIOPort  Port=6  Side=Left
  Tilt Frame : PMIOPort  Port=7  Side=Left
  Out Bus Element : Outport  PortName=m  Element=Tilt
  Out Bus Element1 : Outport  PortName=m  Element=Shift
  Out Bus Element3 : Outport  PortName=m  Element=Blade
  wires:
  BusElementIn1/1 -> Shift Actuator/1(p)
  BusElementIn/1 -> Tilt Actuator/1(p)
  Tilt Actuator/1(m) -> Out Bus Element/1
  Shift Actuator/1(m) -> Out Bus Element1/1
  Constant1/1 -> Switch/1
  BusElementIn2/1 -> Switch/2
  Switch/1 -> Simulink-PS Converter2/1
  Constant/1 -> Switch/3
  Blade/1(m) -> Out Bus Element3/1
  connections:
  Prismatic Blade Shift/LConn1 -- BladeTilt/RConn2
  G/RConn1 -- Blade/LConn3
  Tilt Actuator/RConn1 -- BladeTilt/LConn1
  Tilt Frame/RConn1 -- Tilt Frame1/RConn1 -- Revolute Blade Tilt/LConn1
  BladeTilt/RConn1 -- Shift Actuator/LConn2
  Shift Actuator/RConn1 -- Blade/LConn1
  Prismatic Blade Shift/RConn1 -- Blade/LConn2
  Tilt Actuator/LConn2 -- Tilt Cyl/RConn1
  Revolute Blade Tilt/RConn1 -- BladeTilt/LConn2
  Tilt Actuator/LConn1 -- Tilt/RConn1
  Side/RConn1 -- Shift Actuator/LConn1
  Six DOF Blade Ground/RConn1 -- Blade/LConn5
  World Frame/RConn1 -- Six DOF Blade Ground/LConn1
  Simulink-PS Converter2/RConn1 -- Six DOF Blade Ground/LConn2
  Gbl/RConn1 -- Blade/LConn4

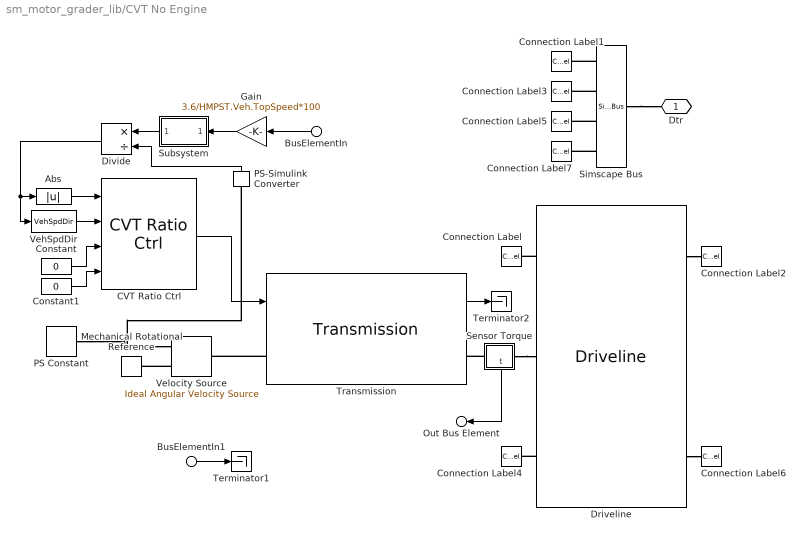
== system sm_motor_grader_lib/CVT No Engine ==
  BusElementIn : Inport  PortName=Cmd  Element=vVeh
  BusElementIn1 : Inport  Port=2  PortName=m  Element=FrameR.Body.Ref.vx
  Abs : Abs  ZeroCross=off  SaturateOnIntegerOverflow=off
  CVT Ratio Ctrl : cvt_powertrain_lib/Controller/CVT Ratio Ctrl  SystemSampleTime=-1  VariantActivationTime=update diagram  EmptyChoice=off  PassThrough=off  PassThroughVariantControl=(default)  EmptyChoiceVariantControl=(default)  AllowFlexibleInterface=on  Latency=0  AutoFrameSizeCalculation=off
  Connection Label : ConnectionLabel  Label=FL
  Connection Label1 : ConnectionLabel  Label=FL
  Connection Label2 : ConnectionLabel  Label=FR
  Connection Label3 : ConnectionLabel  Label=FR
  Connection Label4 : ConnectionLabel  Label=RL
  Connection Label5 : ConnectionLabel  Label=RL
  Connection Label6 : ConnectionLabel  Label=RR
  Connection Label7 : ConnectionLabel  Label=RR
  Constant : Constant  Value=0
  Constant1 : Constant  Value=0
  Divide : Product  Inputs=*/
  Driveline : cvt_powertrain_lib/Driveline  SystemSampleTime=-1  VariantActivationTime=update diagram  EmptyChoice=off  PassThrough=off  PassThroughVariantControl=(default)  EmptyChoiceVariantControl=(default)  AllowFlexibleInterface=on  Latency=0  AutoFrameSizeCalculation=off
  Gain : Gain  Gain=3.6/HMPST.Veh.TopSpeed*100
  Mechanical Rotational Reference : fl_lib/Mechanical/Rotational Elements/Mechanical Rotational Reference
  PS Constant : fl_lib/Physical Signals/Sources/PS Constant  constant=2200 rpm
  PS-Simulink Converter : nesl_utility/PS-Simulink Converter  PhysicalDomain=network_engine_domain  SubClassName=ps_output  LeftPortType=input  RightPortType=output  PseudoPeriodic=off  Frequencies=[]  VectorFormat=inherit  Unit=inherit  AffineConversion=off
  Sensor Torque : Subsystem
      settings: PortSchema="{\"entries\":[{\"content\":{\"sides\":[{\"content\":{\"connectorIds\":[\"LConn1\"]},\"type\":\"ConnectorPlacement.EquallySpacedRectSide\",\"uuid\":\"a60d8853-0bb2-4825-9501-bfce82d3c60b\"},{\"content\":{\"connectorIds\":[\"RConn1\"],\"side\":\"RIGHT\"},\"type\":\"ConnectorPlacement.EquallySpacedRectSide\",\"uuid\":\"bc615e16-29ec-4d17-bdbf-fc0a9930581d\"},{\"content\":{\"side\":\"TOP\"},\"type\":\"ConnectorPlacement.EquallySpacedRectSide\",\"uuid\":\"1f9f0795-d12a-4ada-b455-20f032b748e6\"},{\"content\":{\"connectorIds\":[\"Out1\"],\"side\":\"BOTTOM\"},\"type\":\"ConnectorPlacement.EquallySpacedRectSide\",\"uuid\":\"dcc458f5-a06d-4b01-92f9-dba15bc9e25d\"}]},\"type\":\"ConnectorPlacement.EquallySpacedConnector\",\"uuid\":\"98537a4a-3fd1-4592-a4bd-be27ee472ad2\"}],\"packageUris\":[\"http://schema.mathworks.com/mf0/Connector/R2020b\"],\"version\":\"1.0\"}"
  Simscape Bus : SimscapeBus  HierarchyStrings=RFL;RFR;RRL;RRR
  Subsystem : Subsystem
  Terminator1 : Terminator
  Terminator2 : Terminator
  Transmission : cvt_powertrain_lib_vnts/Transmission  SystemSampleTime=-1  VariantControl=Choice  LabelModeActiveChoice=Electrical  VariantActivationTime=update diagram  EmptyChoice=off  PassThrough=off  PassThroughVariantControl=(default)  EmptyChoiceVariantControl=(default)  AllowFlexibleInterface=on  Latency=0  AutoFrameSizeCalculation=off
      settings: AttributesFormatString=%<LabelModeActiveChoice>
  VehSpdDir : cvt_powertrain_lib/Controller/Desired Ratio Calc/VehSpdDir  SystemSampleTime=-1  VariantActivationTime=update diagram  EmptyChoice=off  PassThrough=off  PassThroughVariantControl=(default)  EmptyChoiceVariantControl=(default)  AllowFlexibleInterface=on  Latency=0  AutoFrameSizeCalculation=off
  Velocity Source : fl_lib/Mechanical/Mechanical Sources/Ideal Angular Velocity Source
  Dtr : PMIOPort  Side=Right
  Out Bus Element : Outport  PortName=meas  Element=trqDrv
  wires:
  Gain/1 -> Subsystem/1(Cmd)
  VehSpdDir/1 -> CVT Ratio Ctrl/2
  Constant/1 -> CVT Ratio Ctrl/3
  Divide/1 -> VehSpdDir/1, Abs/1
  Constant1/1 -> CVT Ratio Ctrl/4
  Abs/1 -> CVT Ratio Ctrl/1
  PS-Simulink Converter/1 -> Divide/2
  Subsystem/1(Out1) -> Divide/1
  CVT Ratio Ctrl/1 -> Transmission/1
  BusElementIn/1 -> Gain/1
  Sensor Torque/1(t) -> Out Bus Element/1
  Transmission/1 -> Terminator2/1
  BusElementIn1/1 -> Terminator1/1
  connections:
  PS-Simulink Converter/LConn1 -- PS Constant/RConn1 -- Velocity Source/RConn1
  Velocity Source/RConn2 -- Mechanical Rotational Reference/LConn1
  Sensor Torque/RConn1 -- Driveline/LConn2
  Sensor Torque/LConn1 -- Transmission/RConn1
  Simscape Bus/RConn1 -- Dtr/RConn1
  Driveline/RConn1 -- Connection Label6/LConn1
  Simscape Bus/LConn3 -- Connection Label5/LConn1
  Driveline/LConn3 -- Connection Label/LConn1
  Simscape Bus/LConn2 -- Connection Label3/LConn1
  Simscape Bus/LConn1 -- Connection Label1/LConn1
  Driveline/RConn3 -- Connection Label2/LConn1
  Simscape Bus/LConn4 -- Connection Label7/LConn1
  Driveline/LConn1 -- Connection Label4/LConn1
  Transmission/LConn1 -- Velocity Source/LConn1

== system sm_motor_grader_lib/Circle ==
  CircleFrameSolid : sm_lib/Body Elements/File Solid  ExtGeomFileName=CircleFrame.step  UnitType=FromFile  ExtGeomFileUnits=m  StepReaderType=HEX  ExportConvexHullGeometry=off  InertiaType=CalculateFromGeometry  BasedOnType=Mass  Density=1000  DensityUnits=kg/m^3  Mass=motGradParams.circleFrame.mass  MassUnits=kg  CenterOfMass=[0 0 0]  CenterOfMassUnits=m  MomentsOfInertia=[1 1 1]  MomentsOfInertiaUnits=kg*m^2  ProductsOfInertia=[0 0 0]  ProductsOfInertiaUnits=kg*m^2  GraphicType=FromGeometry  MarkerShape=Sphere  MarkerSize=10  GraphicVisPropType=SimpleVisualProperties  GraphicDiffuseColor=mtrgrd.clr.circle  GraphicOpacity=1  GraphicSpecularColor=[0.5 0.5 0.5 1.0]  GraphicAmbientColor=[0.15 0.15 0.15 1.0]  GraphicEmissiveColor=[0.0 0.0 0.0 1.0]  GraphicShininess=75  DoExposeReferenceFrame=off  SerializedFrames=<Frames><Frame><Id>Frame1</Id><Value><Name>Drawbar</Name><Origin><Source>GeometricFeature</Source><FeatureName>circular curve 28</FeatureName></Origin><PrimaryAxis><DefinedDirection>+Z</DefinedDirection><Source>ReferenceFrame</Source><SourceDirection>+Z</SourceDirection><FeatureName></FeatureName></PrimaryAxis><SecondaryAxis><DefinedDirection>+X</DefinedDirection><Source>ReferenceFrame</Source><SourceDirection>+X</SourceDirection><FeatureName></FeatureName></SecondaryAxis></Value></Frame><Frame><Id>Frame2</Id><Value><Name>BladeTiltFrame</Name><Origin><Source>GeometricFeature</Source><FeatureName>circular curve 62</FeatureName></Origin><PrimaryAxis><DefinedDirection>-Z</DefinedDirection><Source>GeometricFeature</Source><SourceDirection>+Z</SourceDirection><FeatureName>segment 76</FeatureName></PrimaryAxis><SecondaryAxis><DefinedDirection>+X</DefinedDirection><Source>GeometricFeature</Source><SourceDirection>+X</SourceDirection><FeatureName>segment 73</FeatureName></SecondaryAxis></Value></Frame><Frame><Id>Frame3</Id><Value><Name>BladeTiltCyl</Name><Origin><Source>GeometricFeature</Source><FeatureName>circular curve 37</FeatureName></Origin><PrimaryAxis><DefinedDirection>+Z</DefinedDirection><Source>GeometricFeature</Source><SourceDirection>+Z</SourceDirection><FeatureName>segment 19</FeatureName></PrimaryAxis><SecondaryAxis><DefinedDirection>+X</DefinedDirection><Source>GeometricFeature</Source><SourceDirection>+X</SourceDirection><FeatureName>segment 73</FeatureName></SecondaryAxis></Value></Frame></Frames>
  Rigid Transform : sm_lib/Frames and Transforms/Rigid Transform  RotationMethod=StandardAxis  FollAlignAxisA=+X  BaseAlignAxisA=+Y  FollAlignAxisB=+Y  BaseAlignAxisB=+Z  RotationStandardAxis=+X  RotationAngle=90  RotationAngleUnits=deg  RotationArbitraryAxis=[0 0 1]  RotationSequenceAxes=FollowerAxes  RotationSequence=XYX  RotationSequenceAngles=[0 0 0]  RotationSequenceAnglesUnits=deg  RotationMatrix=[1 0 0;0 1 0;0 0 1]  Quaternion=[1 0 0 0]  TranslationMethod=None  TranslationCartesianOffset=[0 0 0]  TranslationCartesianOffsetUnits=m  TranslationStandardAxis=+Z  TranslationStandardOffset=0  TranslationStandardOffsetUnits=m  TranslationROffset=0  TranslationROffsetUnits=m  TranslationThetaOffset=0  TranslationThetaOffsetUnits=deg  TranslationZOffset=0  TranslationZOffsetUnits=m
  Drawbar : PMIOPort  Side=Left
  Tilt Frame : PMIOPort  Port=2  Side=Right
  Tilt Cyl : PMIOPort  Port=3  Side=Right
  connections:
  Drawbar/RConn1 -- CircleFrameSolid/LConn1
  Tilt Frame/RConn1 -- CircleFrameSolid/RConn1
  Tilt Cyl/RConn1 -- Rigid Transform/RConn1
  Rigid Transform/LConn1 -- CircleFrameSolid/LConn2

== system sm_motor_grader_lib/Contact ==
  Magic Formula : Subsystem  VariantControl=Magic Formula
      mask Display: image('sm_motor_grader_tire_contact_magicFormula_IMAGE.png')
  Point Cloud : Subsystem  VariantControl=Point Cloud
      mask Display: image('sm_motor_grader_tire_contact_points_IMAGE.png')
  Sphere : Subsystem  VariantControl=Sphere
      mask Display: image('sm_motor_grader_tire_contact_sphere_IMAGE.png')
  R : PMIOPort  Side=Left
  G : PMIOPort  Port=2  Side=Right
  m : Outport
